simulink model "multirate_control_model"  (R2024a)
settings: Solver=FixedStepDiscrete  StartTime=0.0  StopTime=10.0  RelTol=1e-3
libraries: simulink x3, slpidlib x1, pil_lib x1
settings Model: Creator=User  LastModifiedBy=User
settings OptimizationCC: DefaultParameterBehavior=Inlined  UseDivisionForNetSlopeComputation=on  GainParamInheritBuiltInType=on  UseFloatMulNetSlope=on  InlineInvariantSignals=on  PassReuseOutputArgsAs=Individual arguments  ZeroExternalMemoryAtStartup=off  ZeroInternalMemoryAtStartup=off  NoFixptDivByZeroProtection=on  EfficientFloat2IntCast=on  LifeSpan=1  OptimizeBlockOrder=speed  DifferentSizesBufferReuse=on  EfficientTunableParamExpr=on
settings DebuggingCC: ParameterTunabilityLossMsg=error
settings HardwareCC: ProdBitPerInt=16  ProdBitPerPointer=16  ProdBitPerSizeT=16  ProdBitPerPtrDiffT=16  ProdLargestAtomicFloat=None  ProdWordSize=16  ProdHWDeviceType=Atmel->AVR (8-bit)
settings SFSimCC: MATLABDynamicMemAlloc=off
settings RTWCC: Description=Embedded Coder  SystemTargetFile=ert.tlc  TemplateMakefile=ert_default_tmf
settings CodeAppCC: ForceParamTrailComments=on  IgnoreCustomStorageClasses=off  OperatorAnnotations=on  SimulinkDataObjDesc=on  SFDataObjDesc=on  CustomSymbolStrGlobalVar=rt$N$M  CustomSymbolStrType=$N$M  CustomSymbolStrFcn=$N$M$F  CustomSymbolStrMacro=$N$M  InsertBlockDesc=on
settings ERTTargetCC: TargetLangStandard=C99 (ISO)  GenerateSampleERTMain=on  IncludeMdlTerminateFcn=off  CombineSignalStateStructs=on  SupportComplex=off  InlinedParameterPlacement=NonHierarchical  ERTCustomFileTemplate=example_file_process.tlc

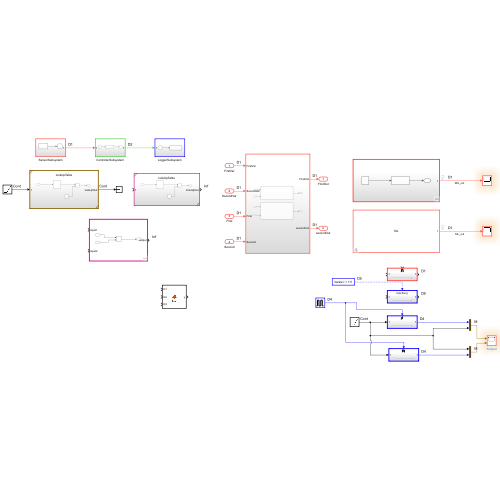
[thumbnail: Simulink's stored preview of the top-level diagram]
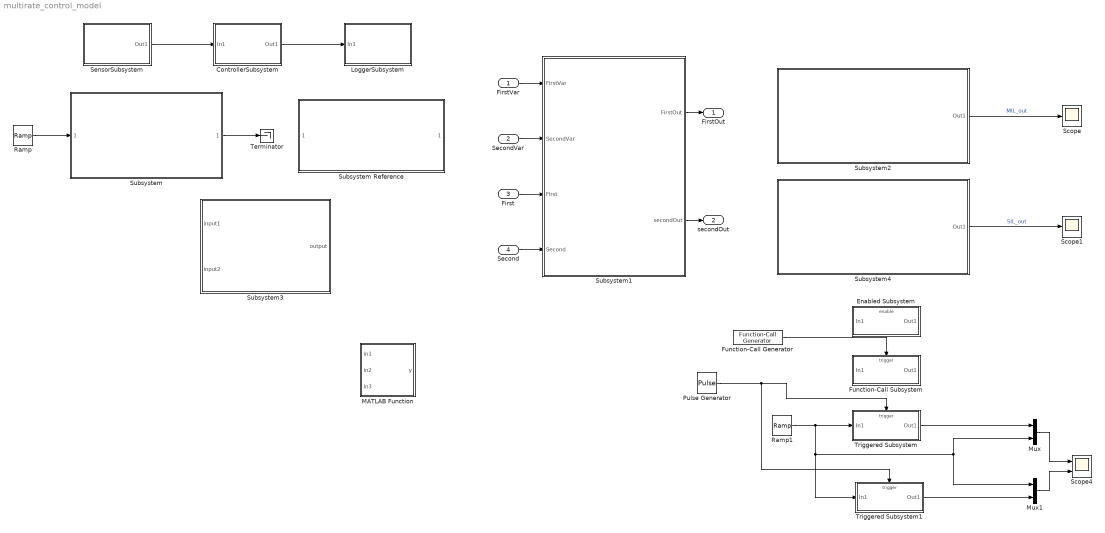
== system multirate_control_model ==
  FirstVar : Inport
  SecondVar : Inport  Port=2
  First : Inport  Port=3
  Second : Inport  Port=4
  ControllerSubsystem : Subsystem
  Enabled Subsystem : Subsystem  TreatAsAtomicUnit=on
  Function-Call Generator : simulink/Ports & Subsystems/Function-Call Generator  sample_time=1  numberOfIterations=5  DisallowWideOutput=off
  Function-Call Subsystem : Subsystem  TreatAsAtomicUnit=on
  LoggerSubsystem : Subsystem
  MATLAB Function : MATLAB Function  TreatAsAtomicUnit=on
  Mux : Mux  Inputs=2
  Mux1 : Mux  Inputs=2
  Pulse Generator : DiscretePulseGenerator  PulseType=Time based  Period=1  PulseWidth=50
  Ramp : simulink/Sources/Ramp  slope=1  start=0  InitialOutput=0
  Ramp1 : simulink/Sources/Ramp  slope=1  start=0  InitialOutput=0
  Scope : Scope
  Scope1 : Scope
  Scope4 : Scope  NumInputPorts=2
  SensorSubsystem : Subsystem
  Subsystem : Subsystem  TreatAsAtomicUnit=on  ReferencedSubsystem=lookUpTable
      settings: RTWFcnNameOpts=Use subsystem name  RTWFileNameOpts=Use subsystem name
  Subsystem Reference : Subsystem  ReferencedSubsystem=lookUpTable
  Subsystem1 : Subsystem  TreatAsAtomicUnit=on
  Subsystem2 : Subsystem  TreatAsAtomicUnit=on  SystemSampleTime=1e-3
  Subsystem3 : Subsystem  TreatAsAtomicUnit=on
  Subsystem4 : Subsystem  Tag=__SL_testing_harness_stub_  DialogController=pil_create_dialog  LoadFcn=|
      | try
      |    if ~strcmp(rtw.pil.getPILVersion, '24.1 (R2024a)_15')
      |       set_param(gcb, 'DialogController', '');
      |       set_param(gcb, 'DialogControllerArgs', '');
      |    end
      | catch e
      |       set_param(gcb, 'DialogController', '');
      |       set_param(gcb, 'DialogControllerArgs', '');
      | end
      mask help: PIL:pil:XILBlockMaskDesc
      mask Display: disp('SIL');
  Terminator : Terminator
  Triggered Subsystem : Subsystem  TreatAsAtomicUnit=on
  Triggered Subsystem1 : Subsystem  TreatAsAtomicUnit=on
  FirstOut : Outport
  secondOut : Outport  Port=2
  wires:
  SensorSubsystem/1(Out1) -> ControllerSubsystem/1(In1)
  ControllerSubsystem/1(Out1) -> LoggerSubsystem/1(In1)
  Ramp/1 -> Subsystem/1
  Subsystem/1 -> Terminator/1
  FirstVar/1 -> Subsystem1/1(FirstVar)
  SecondVar/1 -> Subsystem1/2(SecondVar)
  First/1 -> Subsystem1/3(First)
  Second/1 -> Subsystem1/4(Second)
  Subsystem1/1(FirstOut) -> FirstOut/1
  Subsystem1/2(secondOut) -> secondOut/1
  Subsystem2/1(Out1) -> Scope/1  "MIL_out"
  Subsystem4/1(Out1) -> Scope1/1  "SIL_out"
  Function-Call Generator/1 -> Function-Call Subsystem/Trigger
  Ramp1/1 -> Triggered Subsystem1/1(In1), Mux1/1, Mux/2, Triggered Subsystem/1(In1)
  Pulse Generator/1 -> Triggered Subsystem1/Trigger, Triggered Subsystem/Trigger
  Triggered Subsystem/1(Out1) -> Mux/1
  Triggered Subsystem1/1(Out1) -> Mux1/2
  Mux/1 -> Scope4/1
  Mux1/1 -> Scope4/2

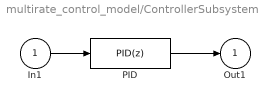
== system multirate_control_model/ControllerSubsystem ==
  In1 : Inport
  PID : slpidlib/PID Controller  Controller=PID  Form=Parallel  TimeDomain=Discrete-time  UseExternalTs=off  SampleTime=-1  IntegratorMethod=Forward Euler  FilterMethod=Forward Euler  ControllerParametersSource=internal  P=1  I=1  UseKiTs=off  D=0  UseExternalDerivativeSource=off  N=100  UseFilter=on  TunerSelectOption=Transfer Function Based (PID Tuner App)  InitialConditionSource=internal  InitialConditionForIntegrator=0  InitialConditionForFilter=0  DifferentiatorICPrevScaledInput=0  ExternalReset=none  TrackingMode=off  Kt=1  LimitOutput=off  SatLimitsSource=internal  UpperSaturationLimit=inf  LowerSaturationLimit=-inf  LinearizeAsGain=off  AntiWindupMode=none  Kb=1  LimitIntegrator=off  UpperIntegratorSaturationLimit=inf  LowerIntegratorSaturationLimit=-inf  POutMin=[]  POutMax=[]  IOutMin=[]  IOutMax=[]  DOutMin=[]  DOutMax=[]  NOutMin=[]  NOutMax=[]  SumOutMin=[]  SumOutMax=[]  SaturationOutMin=[]  SaturationOutMax=[]  PParamMin=[]  PParamMax=[]  IParamMin=[]  IParamMax=[]  DParamMin=[]  DParamMax=[]  NParamMin=[]  NParamMax=[]  KbParamMin=[]  KbParamMax=[]  KtParamMin=[]  KtParamMax=[]  KbOutMin=[]  KbOutMax=[]  KtOutMin=[]  KtOutMax=[]  IntegratorOutMin=[]  IntegratorOutMax=[]  FilterOutMin=[]  FilterOutMax=[]  SumI1OutMin=[]  SumI1OutMax=[]  SumI2OutMin=[]  SumI2OutMax=[]  SumI3OutMin=[]  SumI3OutMax=[]  SumI4OutMin=[]  SumI4OutMax=[]  SumDOutMin=[]  SumDOutMax=[]  DifferentiatorOutMin=[]  DifferentiatorOutMax=[]  FilterDiffOutCoefMin=[]  FilterDiffOutCoefMax=[]  ReciprocalOutMin=[]  ReciprocalOutMax=[]  SumDenOutMin=[]  SumDenOutMax=[]  SumNumOutMin=[]  SumNumOutMax=[]  DivideOutMin=[]  DivideOutMax=[]  UdiffTsProdOutMin=[]  UdiffTsProdOutMax=[]  NTsProdOutMin=[]  NTsProdOutMax=[]  UintegralTsProdOutMin=[]  UintegralTsProdOutMax=[]  UngainTsProdOutMin=[]  UngainTsProdOutMax=[]  ClampingZeroOutDataTypeStr=Inherit: Inherit via back propagation  ClampingZeroOutMin=[]  ClampingZeroOutMax=[]  FilterDenConstantOutDataTypeStr=Inherit: Inherit via back propagation  FilterDenConstantOutMin=[]  FilterDenConstantOutMax=[]  PCopyOutDataTypeStr=Inherit: Inherit via back propagation  PCopyOutMin=[]  PCopyOutMax=[]  NCopyOutDataTypeStr=Inherit: Inherit via back propagation  NCopyOutMin=[]  NCopyOutMax=[]  IntegratorContinuousStateAttributes=''  IntegratorStateMustResolveToSignalObject=off  IntegratorRTWStateStorageClass=Auto  FilterContinuousStateAttributes=''  FilterStateMustResolveToSignalObject=off  FilterRTWStateStorageClass=Auto  ParallelPVariant=InternalParameters  IdealPVariant=Disabled  IVariant=InternalParameters  DVariant=InternalParameters  IntegratorVariant=Discrete  SatVariant=Disabled  AWVariant=Passthrough  PCopyVariant=Disabled  TRVariant=Disabled  FdbkBlocksVariant=Forward  IdealPFdbkVariant=Disabled  SatFdbkVariant=Disabled  DerivativeFilterVariant=ForwardEulerFilter  NVariant=InternalParameters  NCopyVariant=Disabled  FilterICVariant=InternalICsFilter  IntegratorICVariant=InternalICs  ExternalResetVariant=Disabled  TRSumVariant=Passthrough  SumFdbkVariant=Disabled  SumVariant=Sum_PID  TsampFilterVariant=InternalTs  TsampNgainVariant=Passthrough  TsampIntegralVariant=Disabled_SignalSpec  ExternalSaturationOutDataTypeStr=Inherit: Same as second input  DerivativeSourceVariant=ErrorSignal
      settings: LibrarySourceBlock=simulink/Discrete/Discrete PID Controller
  Out1 : Outport
  wires:
  In1/1 -> PID/1
  PID/1 -> Out1/1

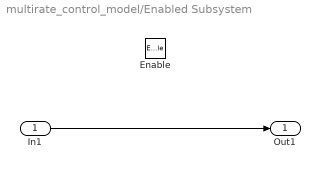
== system multirate_control_model/Enabled Subsystem ==
  In1 : Inport
  Enable : EnablePort
  Out1 : Outport
  wires:
  In1/1 -> Out1/1

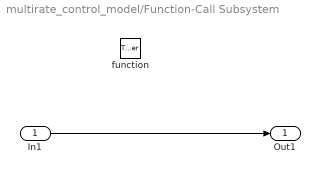
== system multirate_control_model/Function-Call Subsystem ==
  In1 : Inport
  function : TriggerPort  TriggerType=function-call  VariantControl=(inherit)
  Out1 : Outport
  wires:
  In1/1 -> Out1/1

== system multirate_control_model/LoggerSubsystem ==
  In1 : Inport
  Scope : Scope
  wires:
  In1/1 -> Scope/1

== system multirate_control_model/SensorSubsystem ==
  SineWave : Sin  SampleTime=0.001
  Out1 : Outport
  wires:
  SineWave/1 -> Out1/1

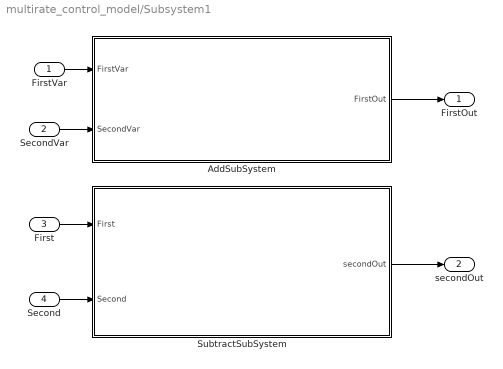
== system multirate_control_model/Subsystem1 ==
  FirstVar : Inport
  SecondVar : Inport  Port=2
  First : Inport  Port=3
  Second : Inport  Port=4
  AddSubSystem : Subsystem  TreatAsAtomicUnit=on
      settings: RTWFcnNameOpts=Use subsystem name  RTWFileNameOpts=Use subsystem name
  SubtractSubSystem : Subsystem
  FirstOut : Outport
  secondOut : Outport  Port=2
  wires:
  Second/1 -> SubtractSubSystem/2(Second)
  SecondVar/1 -> AddSubSystem/2(SecondVar)
  AddSubSystem/1(FirstOut) -> FirstOut/1
  FirstVar/1 -> AddSubSystem/1(FirstVar)
  First/1 -> SubtractSubSystem/1(First)
  SubtractSubSystem/1(secondOut) -> secondOut/1

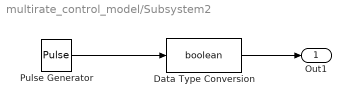
== system multirate_control_model/Subsystem2 ==
  Data Type Conversion : DataTypeConversion  OutDataTypeStr=boolean  SaturateOnIntegerOverflow=off  RndMeth=Floor
  Pulse Generator : DiscretePulseGenerator  Period=2000  PulseWidth=1000  SampleTime=1e-3
  Out1 : Outport  OutDataTypeStr=boolean
  wires:
  Data Type Conversion/1 -> Out1/1
  Pulse Generator/1 -> Data Type Conversion/1

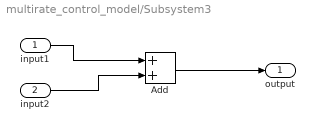
== system multirate_control_model/Subsystem3 ==
  input1 : Inport  OutMin=0  OutMax=255  OutDataTypeStr=uint8  PortDimensions=1
  input2 : Inport  Port=2  OutDataTypeStr=uint8  PortDimensions=1
  Add : Sum
  output : Outport  OutDataTypeStr=uint8  PortDimensions=1
  wires:
  input1/1 -> Add/1
  input2/1 -> Add/2
  Add/1 -> output/1

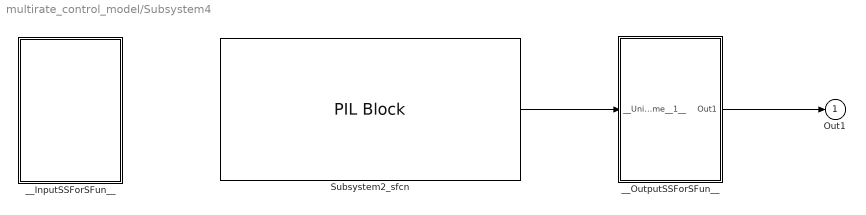
== system multirate_control_model/Subsystem4 ==
  Subsystem2_sfcn : pil_lib/PIL Block  SimulationMode=SIL  IsTopModelPIL=off  CodeDir=Subsystem2_ert_rtw  AnchorDir=D:\ME\Career\04.MBD\Tutorials\SimulinkTut\tut05  ConfigName=Software-in-the-Loop (SIL)  XrelIsTopModelCode=on  XrelIsReusable=off  XrelDWorkNames={}  XrelDWorkTypes={}  XrelModelArgVals={}  XrelOrderedParamNames={}  XRelNonFiniteStyle=NONFINITE_UNUSED  MaskPortLabels=port_label('output',1,'Out1')
  __InputSSForSFun__ : Subsystem
  __OutputSSForSFun__ : Subsystem
  Out1 : Outport  OutDataTypeStr=boolean
  wires:
  __OutputSSForSFun__/1(Out1) -> Out1/1
  Subsystem2_sfcn/1 -> __OutputSSForSFun__/1(__UniqueInportName__1__)

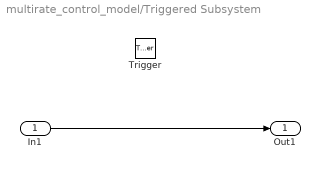
== system multirate_control_model/Triggered Subsystem ==
  In1 : Inport
  Trigger : TriggerPort  VariantControl=(inherit)
  Out1 : Outport
  wires:
  In1/1 -> Out1/1

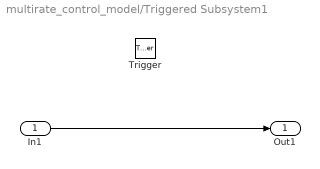
== system multirate_control_model/Triggered Subsystem1 ==
  In1 : Inport
  Trigger : TriggerPort  TriggerType=either  VariantControl=(inherit)
  Out1 : Outport
  wires:
  In1/1 -> Out1/1

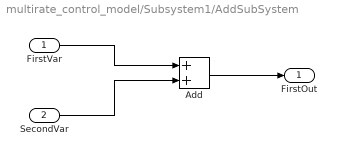
== system multirate_control_model/Subsystem1/AddSubSystem ==
  FirstVar : Inport
  SecondVar : Inport  Port=2
  Add : Sum
  FirstOut : Outport
  wires:
  Add/1 -> FirstOut/1
  SecondVar/1 -> Add/2
  FirstVar/1 -> Add/1

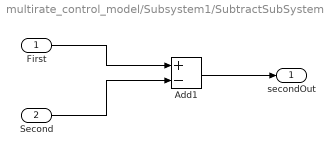
== system multirate_control_model/Subsystem1/SubtractSubSystem ==
  First : Inport
  Second : Inport  Port=2
  Add1 : Sum  Inputs=+-
  secondOut : Outport
  wires:
  First/1 -> Add1/1
  Second/1 -> Add1/2
  Add1/1 -> secondOut/1

== system multirate_control_model/Subsystem4/__InputSSForSFun__ ==

== system multirate_control_model/Subsystem4/__OutputSSForSFun__ ==
  __UniqueInportName__1__ : Inport
  Out1 : Outport  OutDataTypeStr=boolean
  wires:
  __UniqueInportName__1__/1 -> Out1/1

== matlab function multirate_control_model/MATLAB Function ==
  data: in1 input; in2 input; in3 input; y output
function y = fcn(in1,in2, in3)

y = in1+in2+in3;
